simulink model "SupervisoryControlStateMachineTest"  (R2012b)
settings: Solver=ode1  StartTime=0.0  StopTime=Inf  FixedStep=0.001  RelTol=1e-3
PostLoadFcn:
  | , if any(exist('dsrtsu_mdlpostloadfcn', 'file') == [2, 3, 6]), try dsrtsu_mdlpostloadfcn('Execute', bdroot); catch fprintf('Error in PostLoadFcn (dsrtsu_mdlpostloadfcn) for model "%s":\n %s\n', bdroot, lasterr); end, end,
settings Model: DSRTSU_INTERNAL_RTI_VER=430  DSRTSU_INTERNAL_RTI_TYPE=rti1103  DSRTSU_INTERNAL_RTIFPGA=20  BufferReuse=off  Creator=Raghav  LastModifiedBy=Raghav
settings OptimizationCC: BlockReduction=off  OptimizeBlockIOStorage=off  BufferReuse=off  ExpressionFolding=off  LocalBlockOutputs=off
settings HardwareCC: ProdIntDivRoundTo=Zero  ProdEndianess=BigEndian  ProdHWDeviceType=Generic->Custom  TargetIntDivRoundTo=Zero  TargetEndianess=BigEndian  TargetHWDeviceType=Generic->Custom
settings RTWCC: SystemTargetFile=rti1103.tlc  MakeCommand=make_rti  TemplateMakefile=rti1103.tmf  Description=dSPACE DS1103 Hardware Platform  ProcessScript=rti1103_make_rtw_hook
settings STFCustomTargetCC: CodeReplacementLibrary=ANSI_C  ParMdlRefBuildCompliant=on  GeneratePreprocessorConditionals=Disable all  MatFileLogging=on  SystemTargetFile=rti1103.tlc
settings GRTTargetCC: CompOptLevelCompliant=off  ConcurrentExecutionCompliant=off  CombineOutputUpdateFcns=off  GRTInterface=on  ExtModeMexFile=noextcomm

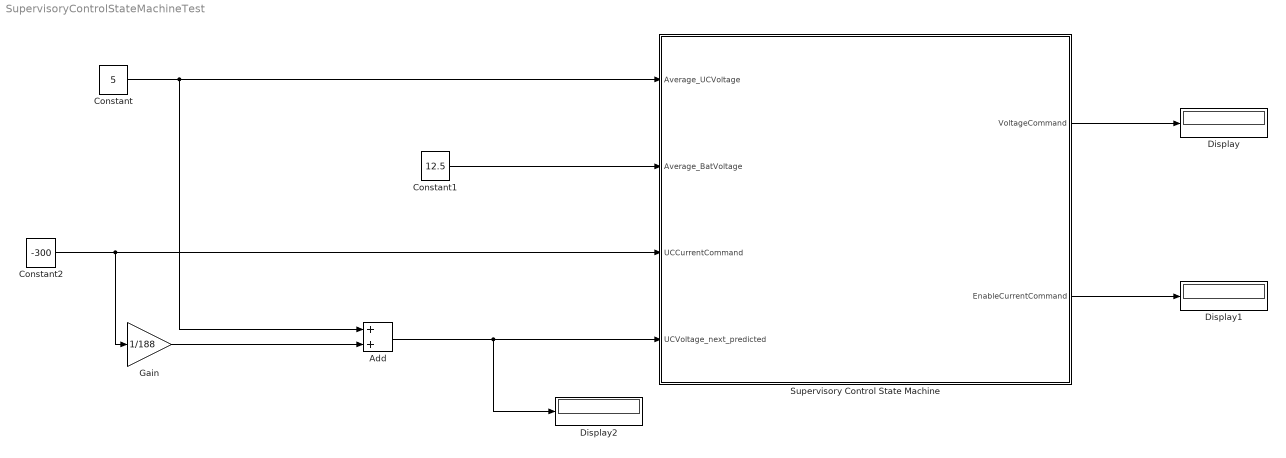
== system SupervisoryControlStateMachineTest ==
  Add : Sum
  Constant : Constant  Value=5
  Constant1 : Constant  Value=12.5
  Constant2 : Constant  Value=-300
  Display : Display
  Display1 : Display
  Display2 : Display
  Gain : Gain  Gain=1/188
  Supervisory Control State Machine : Stateflow chart  TreatAsAtomicUnit=on
  wires:
  Supervisory Control State Machine/1(VoltageCommand) -> Display/1
  Supervisory Control State Machine/2(EnableCurrentCommand) -> Display1/1
  Constant/1 -> Add/1, Supervisory Control State Machine/1(Average_UCVoltage)
  Constant1/1 -> Supervisory Control State Machine/2(Average_BatVoltage)
  Constant2/1 -> Gain/1, Supervisory Control State Machine/3(UCCurrentCommand)
  Gain/1 -> Add/2
  Add/1 -> Display2/1, Supervisory Control State Machine/4(UCVoltage_next_predicted)

== stateflow chart SupervisoryControlStateMachineTest/Supervisory Control State Machine ==
  state InitState
    entry:
    UCVoltageUpperThresh = 7
    UCVoltageLowerThresh = 4
    BatVoltageUpperThresh = 14
    BatVoltageLowerThresh = 11
    delta_Voltage = 0.2
  state ChargeDownState
    during:
    VoltageCommand = UCVoltageUpperThresh - delta_Voltage
    EnableCurrentCommand = 0
  state CurrentControlState
    during:
    EnableCurrentCommand = 1
  state ChargeUpState
    during:
    VoltageCommand = UCVoltageLowerThresh + delta_Voltage
    EnableCurrentCommand = 0
  (default) -> InitState
  InitState -> ChargeDownState [order 2] : [Average_UCVoltage >= UCVoltageUpperThresh ...
      | || UCVoltage_next_predicted >= UCVoltageUpperThresh...
      | || Average_BatVoltage <= BatVoltageLowerThresh]
  InitState -> ChargeUpState [order 1] : [Average_UCVoltage <= UCVoltageLowerThresh ...
      | || UCVoltage_next_predicted <= UCVoltageLowerThresh...
      | || Average_BatVoltage >= BatVoltageUpperThresh]
  InitState -> CurrentControlState [order 3] : [Average_UCVoltage < UCVoltageUpperThresh ...
      | && Average_UCVoltage > UCVoltageLowerThresh ...
      | && Average_BatVoltage > BatVoltageLowerThresh ...
      | && Average_BatVoltage < BatVoltageUpperThresh]
  CurrentControlState -> ChargeDownState [order 1] : [ (Average_UCVoltage >= UCVoltageUpperThresh ...
      | || UCVoltage_next_predicted >= UCVoltageUpperThresh...
      | || Average_BatVoltage <= BatVoltageLowerThresh) ...
      | && UCCurrentCommand >= 0]
  ChargeDownState -> CurrentControlState : [UCCurrentCommand < 0]
  CurrentControlState -> ChargeUpState [order 2] : [ (Average_UCVoltage <= UCVoltageLowerThresh ...
      | || UCVoltage_next_predicted <= UCVoltageLowerThresh...
      | || Average_BatVoltage >= BatVoltageUpperThresh) ...
      | && UCCurrentCommand <= 0]
  ChargeUpState -> CurrentControlState : [UCCurrentCommand > 0]
  data: Average_UCVoltage input; Average_BatVoltage input; UCCurrentCommand input; UCVoltage_next_predicted input; VoltageCommand output double; EnableCurrentCommand output double; BatVoltageLowerThresh local double; BatVoltageUpperThresh local double; UCVoltageLowerThresh local double; UCVoltageUpperThresh local double; delta_Voltage local double
